simulink model "fuzzypid"  (Simulink 7.6)
settings: Solver=ode23tb  StartTime=0.0  StopTime=1  RelTol=1e-3
libraries: powerlib x13, fuzblock x1, powerlib_extras x1
settings Model: Creator=Administrator  LastModifiedBy=Administrator
settings SolverCC: SolverResetMethod=Robust

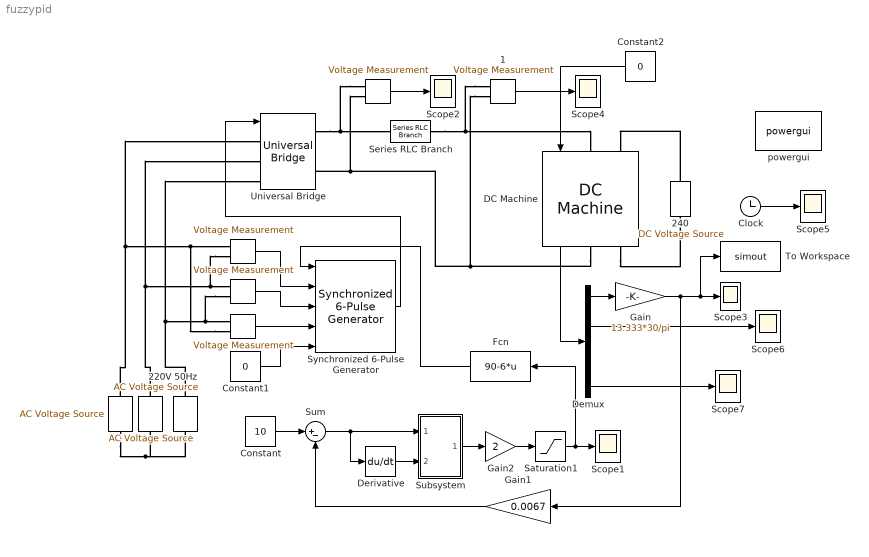
== system fuzzypid ==
  " " : powerlib/Electrical Sources/AC Voltage Source  DialogController=POWERSYS.PowerSysDialog  SystemSampleTime=-1  Amplitude=120*sqrt(3)  Phase=-120  Frequency=50  SampleTime=0  Measurements=None
  "  " : powerlib/Measurements/Voltage Measurement  DialogController=POWERSYS.PowerSysDialog  SystemSampleTime=-1  PhasorSimulation=off  OutputType=Complex  PSBequivalent=0
  "   " : powerlib/Measurements/Voltage Measurement  DialogController=POWERSYS.PowerSysDialog  SystemSampleTime=-1  PhasorSimulation=off  OutputType=Complex  PSBequivalent=0
  "    " : powerlib/Measurements/Voltage Measurement  DialogController=POWERSYS.PowerSysDialog  SystemSampleTime=-1  PhasorSimulation=off  OutputType=Complex  PSBequivalent=0
  "     " : powerlib/Measurements/Voltage Measurement  DialogController=POWERSYS.PowerSysDialog  SystemSampleTime=-1  PhasorSimulation=off  OutputType=Complex  PSBequivalent=0
  "      " : powerlib/Electrical Sources/AC Voltage Source  DialogController=POWERSYS.PowerSysDialog  SystemSampleTime=-1  Amplitude=120*sqrt(3)  Phase=0  Frequency=50  SampleTime=0  Measurements=None
  "     1" : powerlib/Measurements/Voltage Measurement  DialogController=POWERSYS.PowerSysDialog  SystemSampleTime=-1  PhasorSimulation=off  OutputType=Complex  PSBequivalent=0
  220V 50Hz : powerlib/Electrical Sources/AC Voltage Source  DialogController=POWERSYS.PowerSysDialog  SystemSampleTime=-1  Amplitude=120*sqrt(3)  Phase=120  Frequency=50  SampleTime=0  Measurements=None
  240 : powerlib/Electrical Sources/DC Voltage Source  DialogController=POWERSYS.PowerSysDialog  SystemSampleTime=-1  Amplitude=240  Measurements=None
  Clock : Clock
      settings: Decimation=10
  Constant : Constant  Value=10
  Constant1 : Constant  Value=0
  Constant2 : Constant  Value=0
  DC Machine : powerlib/Machines/DC Machine  DialogController=POWERSYS.PowerSysDialog  SystemSampleTime=-1  PresetModel=No  MechanicalLoad=Torque TL  FieldType=Wound  ShowDetailedParameters=on  RLa="[ 0.21  0.00021]"  RLf="[ 146.7  0]"  Laf=0.84  MachineConstant=Torque constant (N.m/A)  Ke=1.8  Kt=1.8  J=0.57  Bm=0  Tf=0  w0=1  Ifinit=1  TsPowergui=0  TsBlock=-1
      settings: AttributesFormatString=\n
  Demux : Demux
  Derivative : Derivative
  Fcn : Fcn  Expr=90-6*u
  Gain : Gain  Gain=13.333*30/pi
  Gain1 : Gain  Gain=0.0067
  Gain2 : Gain  Gain=2
  Saturation1 : Saturate  UpperLimit=10  LowerLimit=-10
  Scope{1..7} (7 alike) : Scope
      Scope1 settings: MaxDataPoints=50000000
      Scope2 settings: SaveName=ScopeData2  MaxDataPoints=50000000
      Scope3 settings: YMin=1925.83  YMax=1925.83  SaveName=n  DataFormat=Array  MaxDataPoints=50000000
      Scope4 settings: YMin=-8  YMax=0.5  SaveName=ScopeData4  MaxDataPoints=50000000
      Scope5 settings: YMin=0.20075  YMax=0.2035  SaveName=ScopeData5  MaxDataPoints=50000000
      Scope6 settings: YMin=226  YMax=233  MaxDataPoints=50000000
      Scope7 settings: YMin=226  YMax=233  SaveName=ScopeData3  MaxDataPoints=50000000
  Series RLC Branch : powerlib/Elements/Series RLC Branch  DialogController=POWERSYS.PowerSysDialog  PhysicalDomain=powersysdomain  SubClassName=unknown  LeftPortType=p1  RightPortType=p1  LConnTagsString=__new0  RConnTagsString=__new0  BranchType=L  Resistance=1  Inductance=0.01  SetiL0=off  InitialCurrent=0  Capacitance=1e-6  Setx0=off  InitialVoltage=0  Measurements=None
  Subsystem : Subsystem
  Sum : Sum  Inputs=|+-
  Synchronized 6-Pulse Generator : powerlib_extras/Control  Blocks/Synchronized 6-Pulse Generator  DialogController=POWERSYS.PowerSysDialog  SystemSampleTime=-1  freq=50  pwidth=10  Double_Pulse=off
  To Workspace : ToWorkspace  VariableName=simout  SampleTime=-1  SaveFormat=Array
  Universal Bridge : powerlib/Power Electronics/Universal Bridge  DialogController=POWERSYS.PowerSysDialog  SystemSampleTime=-1  Arms=3  SnubberResistance=1e5  SnubberCapacitance=inf  Device=Thyristors  Ron=1e-3  Lon=0  ForwardVoltages="[  0  0  ]"  ForwardVoltage=0  GTOparameters=[ 10e-6 , 20e-6 ]  IGBTparameters=[ 1e-6 , 2e-6 ]  Measurements=None  Measurements_2=None  converterType=Rectifier
  powergui : powerlib/powergui  Priority=1  SystemSampleTime=-1  SimulationMode=Continuous  SampleTime=50e-6  frequency=60  SPID=off  DisableSnubberDevices=off  DisableRonSwitches=off  DisableVfSwitches=off  SwTol=0  Interpol=off  frequencyindice=0  echomessages=off  HookPort=off  DisplayEquations=off  FunctionMessages=off  EnableUseOfTLC=off  x0status=blocks  RestoreLinks=warning  ResistiveCurrentMeasurement=off  Ylog=off  Xlog=on  ShowGrid=off  save=off  variable=ZData  ZoomFFT=off  StartTime=0.0  cycles=1  DisplayStyle=1  FreqAxis=off  MaxFrequency=1000  frequencyindicesteady=1  display=off  methode=off
  wires:
  Constant1/1 -> Synchronized 6-Pulse Generator/5
  "    "/1 -> Synchronized 6-Pulse Generator/4
  "   "/1 -> Synchronized 6-Pulse Generator/3
  Synchronized 6-Pulse Generator/1 -> Universal Bridge/1
  "  "/1 -> Synchronized 6-Pulse Generator/2
  DC Machine/1 -> Demux/1
  Demux/1 -> Gain/1
  Gain/1 -> Gain1/1, Scope3/1, To Workspace/1
  Demux/2 -> Scope6/1
  Demux/4 -> Scope7/1
  Constant/1 -> Sum/1
  Gain1/1 -> Sum/2
  Gain2/1 -> Saturation1/1
  Saturation1/1 -> Scope1/1, Fcn/1
  Fcn/1 -> Synchronized 6-Pulse Generator/1
  "     "/1 -> Scope2/1
  "     1"/1 -> Scope4/1
  Clock/1 -> Scope5/1
  Constant2/1 -> DC Machine/1
  Sum/1 -> Subsystem/1(In1), Derivative/1
  Derivative/1 -> Subsystem/2(In2)
  Subsystem/1(Out1) -> Gain2/1
  connections:
  "    "/LConn2 -- "  "/LConn1 -- "      "/RConn1 -- Universal Bridge/LConn1
  "  "/LConn2 -- "   "/LConn1 -- " "/RConn1 -- Universal Bridge/LConn2
  "   "/LConn2 -- "    "/LConn1 -- 220V 50Hz/RConn1 -- Universal Bridge/LConn3
  "     "/LConn1 -- Universal Bridge/RConn1 -- Series RLC Branch/LConn1
  "     1"/LConn1 -- Series RLC Branch/RConn1 -- DC Machine/LConn1
  "     1"/LConn2 -- DC Machine/RConn1 -- Universal Bridge/RConn2 -- "     "/LConn2
  " "/LConn1 -- "      "/LConn1 -- 220V 50Hz/LConn1
  240/RConn1 -- DC Machine/LConn2
  DC Machine/RConn2 -- 240/LConn1

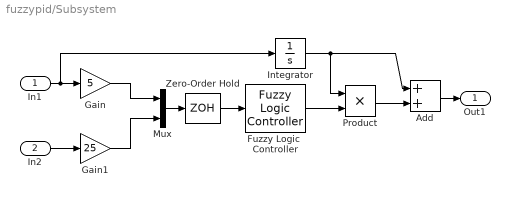
== system fuzzypid/Subsystem ==
  In1 : Inport
  In2 : Inport  Port=2
  Add : Sum
  Fuzzy Logic  Controller : fuzblock/Fuzzy Logic  Controller  SystemSampleTime=-1  fis=FC
  Gain : Gain  Gain=5
  Gain1 : Gain  Gain=25
  Integrator : Integrator
  Mux : Mux  Inputs=2
  Product : Product  RndMeth=Zero
  Zero-Order Hold : ZeroOrderHold
  Out1 : Outport
  wires:
  Gain/1 -> Mux/1
  Gain1/1 -> Mux/2
  Integrator/1 -> Product/1, Add/1
  Fuzzy Logic  Controller/1 -> Product/2
  Product/1 -> Add/2
  In1/1 -> Gain/1, Integrator/1
  In2/1 -> Gain1/1
  Add/1 -> Out1/1
  Mux/1 -> Zero-Order Hold/1
  Zero-Order Hold/1 -> Fuzzy Logic  Controller/1
